simulink model "p1_MPU"  (R2023a)
settings: Solver=FixedStepDiscrete  StartTime=0.0  StopTime=inf  FixedStep=Ts_MPU  RelTol=1e-3  EnableMultiTasking=on
PreLoadFcn:
  | p1_params_new
  | spiDataDefinition
InitFcn:
  | p1_params_new
  | spiDataDefinition
values from neighbouring files (symbols this model uses):
  B = SSest(T,15)+Boffset    [AACplottingcode.m]    (also in Ext_MPCPara.m = SSD.B; IMECE06plottingcode.m = SSest(T,15); If_alpha_tp_observer.m; If_alpha_tp_observer_for_c_code.m)
undefined symbols (not defined in the file or in its folder): DrivetrainLeft, DrivetrainRight, p1data, p1params, Ts_MPU
libraries: simulink x54, raspberrypiBasiclib x8, raspberrypiCommlib x4, embedlinuxNetworklib x2
(part 2 of 2)

== system p1_MPU/Receive Analog Inputs/Switch Case Action Subsystem3 ==
  In1 : Inport
  Action Port : ActionPort  ActionPortLabel=case [ 4 ]:
  Out1 : Outport
  wires:
  In1/1 -> Out1/1

== system p1_MPU/Receive Analog Inputs/Switch Case Action Subsystem4 ==
  In1 : Inport
  Action Port : ActionPort  ActionPortLabel=case [ 6 ]:
  Out1 : Outport
  wires:
  In1/1 -> Out1/1

== system p1_MPU/Receive Analog Inputs/Switch Case Action Subsystem5 ==
  In1 : Inport
  Action Port : ActionPort  ActionPortLabel=case [ 7 ]:
  Out1 : Outport
  wires:
  In1/1 -> Out1/1

== system p1_MPU/Receive Analog Inputs/Switch Case Action Subsystem6 ==
  In1 : Inport
  Action Port : ActionPort  ActionPortLabel=case [ 8 ]:
  Out1 : Outport
  wires:
  In1/1 -> Out1/1

== system p1_MPU/Receive Analog Inputs/Switch Case Action Subsystem7 ==
  In1 : Inport
  Action Port : ActionPort  ActionPortLabel=case [ 9 ]:
  Out1 : Outport
  wires:
  In1/1 -> Out1/1

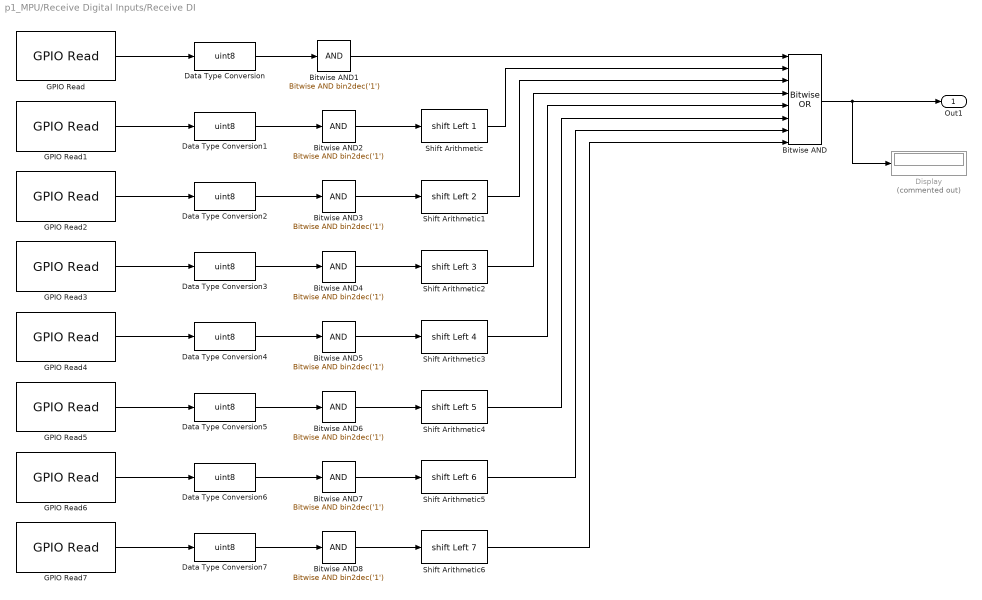
== system p1_MPU/Receive Digital Inputs/Receive DI ==
  Bitwise AND : simulink/Logic and Bit Operations/Bitwise Operator  logicop=OR  UseBitMask=off  NumInputPorts=8  BitMask=bin2dec('11011001')  BitMaskRealWorld=Stored Integer
      settings: LibrarySourceBlock=|
      | simulink/Quick Insert/Logic and Bit
      | Operations/Bitwise AND
  Bitwise AND{1..8} (8 alike) : simulink/Logic and Bit Operations/Bitwise Operator  logicop=AND  UseBitMask=on  BitMask=bin2dec('1')  BitMaskRealWorld=Stored Integer
      settings: LibrarySourceBlock=|
      | simulink/Quick Insert/Logic and Bit
      | Operations/Bitwise AND
  Data Type Conversion{,1..7} (8 alike) : DataTypeConversion  OutDataTypeStr=uint8  SaturateOnIntegerOverflow=off  RndMeth=Floor
  Display : Display  Commented=on
  GPIO Read : raspberrypiBasiclib/GPIO Read  board=Pi 4 Model B  gpio=4  internalResistor=Off  sampleTime=Ts_MPU  direction=Input  blockPlatform=Raspberry Pi
  GPIO Read1 : raspberrypiBasiclib/GPIO Read  board=Pi 4 Model B  gpio=5  internalResistor=Off  sampleTime=Ts_MPU  direction=Input  blockPlatform=Raspberry Pi
  GPIO Read2 : raspberrypiBasiclib/GPIO Read  board=Pi 4 Model B  gpio=6  internalResistor=Off  sampleTime=Ts_MPU  direction=Input  blockPlatform=Raspberry Pi
  GPIO Read3 : raspberrypiBasiclib/GPIO Read  board=Pi 4 Model B  gpio=12  internalResistor=Off  sampleTime=Ts_MPU  direction=Input  blockPlatform=Raspberry Pi
  GPIO Read4 : raspberrypiBasiclib/GPIO Read  board=Pi 4 Model B  gpio=13  internalResistor=Off  sampleTime=Ts_MPU  direction=Input  blockPlatform=Raspberry Pi
  GPIO Read5 : raspberrypiBasiclib/GPIO Read  board=Pi 4 Model B  gpio=16  internalResistor=Off  sampleTime=Ts_MPU  direction=Input  blockPlatform=Raspberry Pi
  GPIO Read6 : raspberrypiBasiclib/GPIO Read  board=Pi 4 Model B  gpio=21  internalResistor=Off  sampleTime=Ts_MPU  direction=Input  blockPlatform=Raspberry Pi
  GPIO Read7 : raspberrypiBasiclib/GPIO Read  board=Pi 4 Model B  gpio=26  internalResistor=Off  sampleTime=Ts_MPU  direction=Input  blockPlatform=Raspberry Pi
  Shift Arithmetic : ArithShift  BitShiftNumber=1  BitShiftDirection=Left
  Shift Arithmetic1 : ArithShift  BitShiftNumber=2  BitShiftDirection=Left
  Shift Arithmetic2 : ArithShift  BitShiftNumber=3  BitShiftDirection=Left
  Shift Arithmetic3 : ArithShift  BitShiftNumber=4  BitShiftDirection=Left
  Shift Arithmetic4 : ArithShift  BitShiftNumber=5  BitShiftDirection=Left
  Shift Arithmetic5 : ArithShift  BitShiftNumber=6  BitShiftDirection=Left
  Shift Arithmetic6 : ArithShift  BitShiftNumber=7  BitShiftDirection=Left
  Out1 : Outport
  wires:
  Shift Arithmetic5/1 -> Bitwise AND/7
  GPIO Read2/1 -> Data Type Conversion2/1
  Shift Arithmetic4/1 -> Bitwise AND/6
  Shift Arithmetic1/1 -> Bitwise AND/3
  Shift Arithmetic3/1 -> Bitwise AND/5
  Shift Arithmetic/1 -> Bitwise AND/2
  Shift Arithmetic2/1 -> Bitwise AND/4
  Shift Arithmetic6/1 -> Bitwise AND/8
  Bitwise AND/1 -> Display/1, Out1/1
  Data Type Conversion/1 -> Bitwise AND1/1
  Data Type Conversion1/1 -> Bitwise AND2/1
  Data Type Conversion2/1 -> Bitwise AND3/1
  Data Type Conversion3/1 -> Bitwise AND4/1
  Data Type Conversion4/1 -> Bitwise AND5/1
  Data Type Conversion5/1 -> Bitwise AND6/1
  Data Type Conversion6/1 -> Bitwise AND7/1
  Data Type Conversion7/1 -> Bitwise AND8/1
  Bitwise AND1/1 -> Bitwise AND/1
  Bitwise AND2/1 -> Shift Arithmetic/1
  Bitwise AND3/1 -> Shift Arithmetic1/1
  Bitwise AND4/1 -> Shift Arithmetic2/1
  Bitwise AND5/1 -> Shift Arithmetic3/1
  Bitwise AND6/1 -> Shift Arithmetic4/1
  Bitwise AND7/1 -> Shift Arithmetic5/1
  Bitwise AND8/1 -> Shift Arithmetic6/1
  GPIO Read/1 -> Data Type Conversion/1
  GPIO Read7/1 -> Data Type Conversion7/1
  GPIO Read6/1 -> Data Type Conversion6/1
  GPIO Read5/1 -> Data Type Conversion5/1
  GPIO Read4/1 -> Data Type Conversion4/1
  GPIO Read3/1 -> Data Type Conversion3/1
  GPIO Read1/1 -> Data Type Conversion1/1

== system p1_MPU/Data Processing/Subsystem/Break Bytes ==
  In1 : Inport
  Data Type Conversion : DataTypeConversion  OutDataTypeStr=uint8  ConvertRealWorld=Stored Integer (SI)  SaturateOnIntegerOverflow=off  RndMeth=Floor
  Data Type Conversion1 : DataTypeConversion  OutDataTypeStr=uint8  ConvertRealWorld=Stored Integer (SI)  SaturateOnIntegerOverflow=off  RndMeth=Floor
  Shift Arithmetic : ArithShift  BitShiftNumber=8  BitShiftDirection=Right
  Out1 : Outport
  Out2 : Outport  Port=2
  wires:
  Data Type Conversion/1 -> Out1/1
  Data Type Conversion1/1 -> Out2/1
  Shift Arithmetic/1 -> Data Type Conversion1/1
  In1/1 -> Data Type Conversion/1, Shift Arithmetic/1

== system p1_MPU/Data Processing/Subsystem/Break Bytes1 ==
  In1 : Inport
  Data Type Conversion : DataTypeConversion  OutDataTypeStr=uint8  ConvertRealWorld=Stored Integer (SI)  SaturateOnIntegerOverflow=off  RndMeth=Floor
  Data Type Conversion1 : DataTypeConversion  OutDataTypeStr=uint8  ConvertRealWorld=Stored Integer (SI)  SaturateOnIntegerOverflow=off  RndMeth=Floor
  Shift Arithmetic : ArithShift  BitShiftNumber=8  BitShiftDirection=Right
  Out1 : Outport
  Out2 : Outport  Port=2
  wires:
  In1/1 -> Shift Arithmetic/1, Data Type Conversion/1
  Shift Arithmetic/1 -> Data Type Conversion1/1
  Data Type Conversion1/1 -> Out2/1
  Data Type Conversion/1 -> Out1/1

== system p1_MPU/Data Processing/Subsystem/Break Bytes2 ==
  In1 : Inport
  Data Type Conversion : DataTypeConversion  OutDataTypeStr=uint8  ConvertRealWorld=Stored Integer (SI)  SaturateOnIntegerOverflow=off  RndMeth=Floor
  Data Type Conversion1 : DataTypeConversion  OutDataTypeStr=uint8  ConvertRealWorld=Stored Integer (SI)  SaturateOnIntegerOverflow=off  RndMeth=Floor
  Shift Arithmetic : ArithShift  BitShiftNumber=8  BitShiftDirection=Right
  Out1 : Outport
  Out2 : Outport  Port=2
  wires:
  Data Type Conversion/1 -> Out1/1
  Data Type Conversion1/1 -> Out2/1
  Shift Arithmetic/1 -> Data Type Conversion1/1
  In1/1 -> Data Type Conversion/1, Shift Arithmetic/1

== system p1_MPU/Data Processing/Subsystem/Break Bytes3 ==
  In1 : Inport
  Data Type Conversion : DataTypeConversion  OutDataTypeStr=uint8  ConvertRealWorld=Stored Integer (SI)  SaturateOnIntegerOverflow=off  RndMeth=Floor
  Data Type Conversion1 : DataTypeConversion  OutDataTypeStr=uint8  ConvertRealWorld=Stored Integer (SI)  SaturateOnIntegerOverflow=off  RndMeth=Floor
  Shift Arithmetic : ArithShift  BitShiftNumber=8  BitShiftDirection=Right
  Out1 : Outport
  Out2 : Outport  Port=2
  wires:
  In1/1 -> Shift Arithmetic/1, Data Type Conversion/1
  Shift Arithmetic/1 -> Data Type Conversion1/1
  Data Type Conversion1/1 -> Out2/1
  Data Type Conversion/1 -> Out1/1

== system p1_MPU/Data Processing/Subsystem/Break Bytes4 ==
  In1 : Inport
  Data Type Conversion : DataTypeConversion  OutDataTypeStr=uint8  ConvertRealWorld=Stored Integer (SI)  SaturateOnIntegerOverflow=off  RndMeth=Floor
  Data Type Conversion1 : DataTypeConversion  OutDataTypeStr=uint8  ConvertRealWorld=Stored Integer (SI)  SaturateOnIntegerOverflow=off  RndMeth=Floor
  Shift Arithmetic : ArithShift  BitShiftNumber=8  BitShiftDirection=Right
  Out1 : Outport
  Out2 : Outport  Port=2
  wires:
  Data Type Conversion/1 -> Out1/1
  Data Type Conversion1/1 -> Out2/1
  Shift Arithmetic/1 -> Data Type Conversion1/1
  In1/1 -> Data Type Conversion/1, Shift Arithmetic/1

== system p1_MPU/Data Processing/Subsystem/Break Bytes5 ==
  In1 : Inport
  Data Type Conversion : DataTypeConversion  OutDataTypeStr=uint8  ConvertRealWorld=Stored Integer (SI)  SaturateOnIntegerOverflow=off  RndMeth=Floor
  Data Type Conversion1 : DataTypeConversion  OutDataTypeStr=uint8  ConvertRealWorld=Stored Integer (SI)  SaturateOnIntegerOverflow=off  RndMeth=Floor
  Shift Arithmetic : ArithShift  BitShiftNumber=8  BitShiftDirection=Right
  Out1 : Outport
  Out2 : Outport  Port=2
  wires:
  In1/1 -> Shift Arithmetic/1, Data Type Conversion/1
  Shift Arithmetic/1 -> Data Type Conversion1/1
  Data Type Conversion1/1 -> Out2/1
  Data Type Conversion/1 -> Out1/1

== system p1_MPU/Data Processing/Subsystem/Break Bytes6 ==
  In1 : Inport
  Data Type Conversion : DataTypeConversion  OutDataTypeStr=uint8  ConvertRealWorld=Stored Integer (SI)  SaturateOnIntegerOverflow=off  RndMeth=Floor
  Data Type Conversion1 : DataTypeConversion  OutDataTypeStr=uint8  ConvertRealWorld=Stored Integer (SI)  SaturateOnIntegerOverflow=off  RndMeth=Floor
  Shift Arithmetic : ArithShift  BitShiftNumber=8  BitShiftDirection=Right
  Out1 : Outport
  Out2 : Outport  Port=2
  wires:
  Data Type Conversion/1 -> Out1/1
  Data Type Conversion1/1 -> Out2/1
  Shift Arithmetic/1 -> Data Type Conversion1/1
  In1/1 -> Data Type Conversion/1, Shift Arithmetic/1

== system p1_MPU/Data Processing/Subsystem/Break Bytes7 ==
  In1 : Inport
  Data Type Conversion : DataTypeConversion  OutDataTypeStr=uint8  ConvertRealWorld=Stored Integer (SI)  SaturateOnIntegerOverflow=off  RndMeth=Floor
  Data Type Conversion1 : DataTypeConversion  OutDataTypeStr=uint8  ConvertRealWorld=Stored Integer (SI)  SaturateOnIntegerOverflow=off  RndMeth=Floor
  Shift Arithmetic : ArithShift  BitShiftNumber=8  BitShiftDirection=Right
  Out1 : Outport
  Out2 : Outport  Port=2
  wires:
  In1/1 -> Shift Arithmetic/1, Data Type Conversion/1
  Shift Arithmetic/1 -> Data Type Conversion1/1
  Data Type Conversion1/1 -> Out2/1
  Data Type Conversion/1 -> Out1/1
